simulink model "RobotModel"  (R2017a)
settings: Solver=ode3  StartTime=0.0  StopTime=10.0  FixedStep=0.01  RelTol=1e-3  EnableMultiTasking=on
settings Model: Creator=ejlobato  LastModifiedBy=Henry
settings DataIOCC: LimitDataPoints=on  SaveFormat=Array
settings OptimizationCC: ExpressionDepthLimit=2147483647  LifeSpan=inf
settings DebuggingCC: UnderspecifiedInitializationDetection=Classic  MergeDetectMultiDrivingBlocksExec=none  SolverPrmCheckMsg=warning  StateNameClashWarn=warning  SFUnexpectedBacktrackingDiag=warning  SFNoUnconditionalDefaultTransitionDiag=warning  SFExecutionAtInitializationDiag=none
settings HardwareCC: ProdBitPerPointer=32  ProdBitPerSizeT=32  ProdBitPerPtrDiffT=32  ProdLargestAtomicFloat=None  ProdIntDivRoundTo=Undefined  ProdEndianess=Unspecified  ProdWordSize=32  ProdHWDeviceType=32-bit Generic
settings ModelReferenceCC: PropagateSignalLabelsOutOfModel=off
settings GRTTargetCC: TargetLangStandard=C89/C90 (ANSI)  GeneratePreprocessorConditionals=Disable all
settings ConfigComp: CovMetricSettings=dw  CovHtmlReporting=on  CovSaveCumulativeToWorkspaceVar=on  CovSaveSingleToWorkspaceVar=on  CovExternalEMLEnable=off

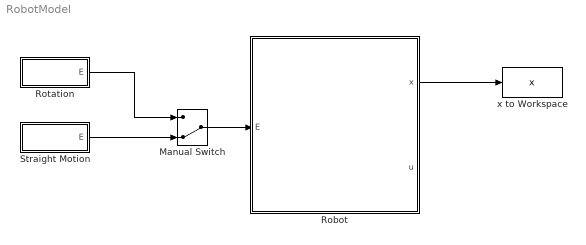
== system RobotModel ==
  Manual Switch : ManualSwitch  CurrentSetting=0
  Robot : Subsystem  mask{xIni=0, yIni=0, aIni=0, uIni=0, vIni=0, wIni=0}
      mask prompts: xIni "Enter xIni"; yIni "Enter yIni"; aIni "Enter aIni"; uIni "Enter uIni"; vIni "Enter vIni"; wIni "Enter wIni"
      mask help:
      | Users must specify the initial position and orientation (xIni,yIni,aIni),
      | and the initial velocities (uIni,vIni,wIni) in the body frame.
      mask Display: image(imread('WolfBot.png'))
  Rotation : Subsystem
  Straight Motion : Subsystem
  x to Workspace : ToWorkspace  VariableName=x  SaveFormat=Timeseries  SampleTime=-1
  wires:
  Straight Motion/1(E) -> Manual Switch/2
  Manual Switch/1 -> Robot/1(E)
  Rotation/1(E) -> Manual Switch/1
  Robot/1(x) -> x to Workspace/1

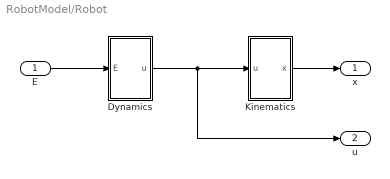
== system RobotModel/Robot ==
  E : Inport
  Dynamics : Subsystem
  Kinematics : Subsystem
  x : Outport
  u : Outport  Port=2
  wires:
  Dynamics/1(u) -> u/1, Kinematics/1(u)
  E/1 -> Dynamics/1(E)
  Kinematics/1(x) -> x/1

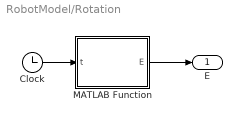
== system RobotModel/Rotation ==
  Clock : Clock
  MATLAB Function : MATLAB Function  TreatAsAtomicUnit=on
  E : Outport
  wires:
  MATLAB Function/1(E) -> E/1
  Clock/1 -> MATLAB Function/1(t)

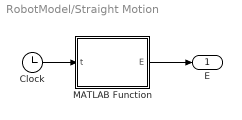
== system RobotModel/Straight Motion ==
  Clock : Clock
  MATLAB Function : MATLAB Function  TreatAsAtomicUnit=on
  E : Outport
  wires:
  MATLAB Function/1(E) -> E/1
  Clock/1 -> MATLAB Function/1(t)

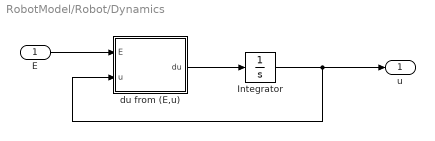
== system RobotModel/Robot/Dynamics ==
  E : Inport  PortDimensions=3
  Integrator : Integrator  InitialCondition=[uIni vIni wIni]
  du from (E,u) : MATLAB Function  TreatAsAtomicUnit=on
  u : Outport
  wires:
  Integrator/1 -> u/1, du from (E,u)/2(u)
  du from (E,u)/1(du) -> Integrator/1
  E/1 -> du from (E,u)/1(E)

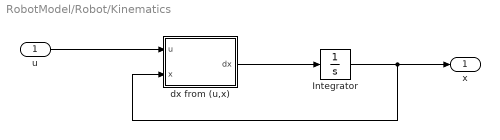
== system RobotModel/Robot/Kinematics ==
  u : Inport  PortDimensions=3
  Integrator : Integrator  InitialCondition=[xIni yIni aIni]
  dx from (u,x) : MATLAB Function  TreatAsAtomicUnit=on
  x : Outport
  wires:
  Integrator/1 -> x/1, dx from (u,x)/2(x)
  u/1 -> dx from (u,x)/1(u)
  dx from (u,x)/1(dx) -> Integrator/1

== matlab function RobotModel/Robot/Dynamics/du from (E,u) ==
  data: E input; u input; du output
function du = fcn(E,u)
% This function returns the derivative of the velocity as a function of the
% voltage input and current velocity. This implements the forward
% dynamics.

m=1.5;
Iz=0.0059;
R=0.0254;
L=0.0889;
n=100;
Ra=16.66;
k2=0.002361;
k3=0.004244;
b0=1.2777e-6;
J0=1.2581e-9;

H = [1/m,0,0; 0,1/m,0; 0,0,1/Iz];
B = [0,cos(pi/6),-cos(pi/6); -1,sin(pi/6),sin(pi/6); L,L,L];
G = eye([3,3]) + H*B*transpose(B)*(((n^2)*J0)/(R^2));

du = inv(G)*[u(3)*u(2); -u(3)*u(1); 0] -inv(G)*H*B*transpose(B)*((k2*k3)/Ra + b0)*(n^2/R^2)*u + inv(G)*H*B*((k2*n)/(R*Ra))*E;

== matlab function RobotModel/Robot/Kinematics/dx from (u,x) ==
  data: u input; dx output; x input
function dx = fcn(u,x)
% This function computes the derivative of the position and orientation as
% a function of the velocity and current position.
m=1.5;
Iz=0.0059;
R=0.0254;
L=0.0889;
n=100;
Ra=16.66;
k2=0.002361;
k3=0.004244;
b0=1.2777e-6;
J0=1.2581e-9;

dx = [cos(x(3)),-sin(x(3)),0; sin(x(3)),cos(x(3)),0; 0,0,1] * u;

== matlab function RobotModel/Rotation/MATLAB Function ==
  data: E output; t input
function E = fcn(t)
% Voltage input

E = [3; 3; 3];

== matlab function RobotModel/Straight Motion/MATLAB Function ==
  data: E output; t input
function E = fcn(t)
% Desired voltage input.

E = [0; 3; -3];
